simulink model "Ball_Fre"  (R2020b)
settings: Solver=VariableStepAuto  StartTime=0.0  StopTime=10.0  RelTol=1e-3
settings Model: Creator=huang  LastModifiedBy=huang

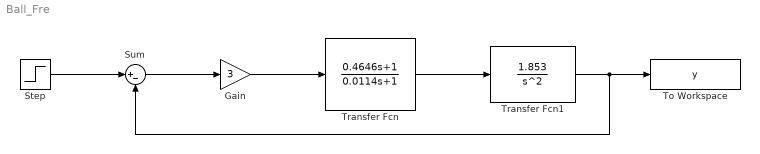
== system Ball_Fre ==
  Gain : Gain  Gain=3
  Step : Step  SampleTime=0
  Sum : Sum  Inputs=|+-
  To Workspace : ToWorkspace  VariableName=y  SampleTime=-1
  Transfer Fcn : TransferFcn  Numerator=[0.4646 1]  Denominator=[0.0114 1]
  Transfer Fcn1 : TransferFcn  Numerator=1.853  Denominator=[1 0 0]
  wires:
  Transfer Fcn/1 -> Transfer Fcn1/1
  Gain/1 -> Transfer Fcn/1
  Sum/1 -> Gain/1
  Transfer Fcn1/1 -> Sum/2, To Workspace/1
  Step/1 -> Sum/1
